simulink model "nonlinearAirframe"  (R2018a)
settings: Solver=ode3  StartTime=0  StopTime=10.0  FixedStep=Ts  RelTol=1e-3  EnableMultiTasking=on
undefined symbols (not defined in the file): e_m_X, e_m_Y, e_p_X, e_p_Y, Earth, initPosLLA, k_ac_X, k_ac_Y, k_as_X, k_as_Y, k_ra_X, k_ra_Y, k_rs_X, k_rs_Y, r_m_X, r_m_Y, r_sm_X, r_sm_Y, Vehicle, WGS84
libraries: actuatorsLibrary x3, shared6dof x1, aerolibtransform2 x1
settings Model: Creator=The MathWorks, Inc.  LastModifiedBy=Ducted Fan
settings SolverCC: AutoInsertRateTranBlk=on
settings DataIOCC: SaveFormat=Array  SaveOutput=off  SignalLogging=off  DSMLogging=off  SaveTime=off
settings OptimizationCC: BlockReduction=off  DefaultParameterBehavior=Inlined  BufferReuse=off  LifeSpan=inf
settings DebuggingCC: AlgebraicLoopMsg=none  UnderspecifiedInitializationDetection=Classic  MergeDetectMultiDrivingBlocksExec=none  UnconnectedInputMsg=none  UnconnectedOutputMsg=none  UnconnectedLineMsg=none  AllowSymbolicDim=off  SFUnexpectedBacktrackingDiag=warning  SFNoUnconditionalDefaultTransitionDiag=warning  SFExecutionAtInitializationDiag=none
settings HardwareCC: ProdBitPerPointer=32  ProdBitPerSizeT=32  ProdBitPerPtrDiffT=32  ProdLargestAtomicFloat=None  ProdIntDivRoundTo=Undefined  ProdEndianess=Unspecified  ProdWordSize=32  ProdHWDeviceType=32-bit Generic
settings ModelReferenceCC: PropagateSignalLabelsOutOfModel=off
settings CodeAppCC: StateflowObjectComments=on
settings GRTTargetCC: TargetLangStandard=C89/C90 (ANSI)  GeneratePreprocessorConditionals=Disable all
settings ConfigComp: CovMetricSettings=dw  CovHtmlReporting=on  CovSaveCumulativeToWorkspaceVar=on  CovSaveSingleToWorkspaceVar=on  CovExternalEMLEnable=off  CovSFcnEnable=off

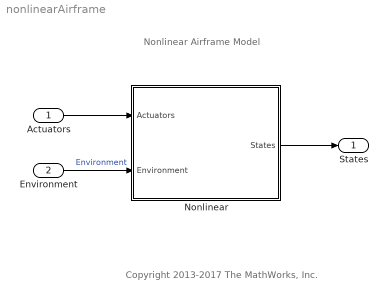
== system nonlinearAirframe ==
  note: Copyright 2013-2017 The MathWorks, Inc.
  note: Nonlinear Airframe Model
  Actuators : Inport  OutDataTypeStr=Bus: ActuatorsBus
  Environment : Inport  Port=2  OutDataTypeStr=Bus: EnvironmentBus  BusOutputAsStruct=on
  Nonlinear : Subsystem  TreatAsAtomicUnit=on
      mask init:
      | vehicleNonlinearVars;
  States : Outport  OutDataTypeStr=Bus: StatesBus  BusOutputAsStruct=on
  wires:
  Actuators/1 -> Nonlinear/1(Actuators)
  Environment/1 -> Nonlinear/2(Environment)  "Environment"
  Nonlinear/1(States) -> States/1

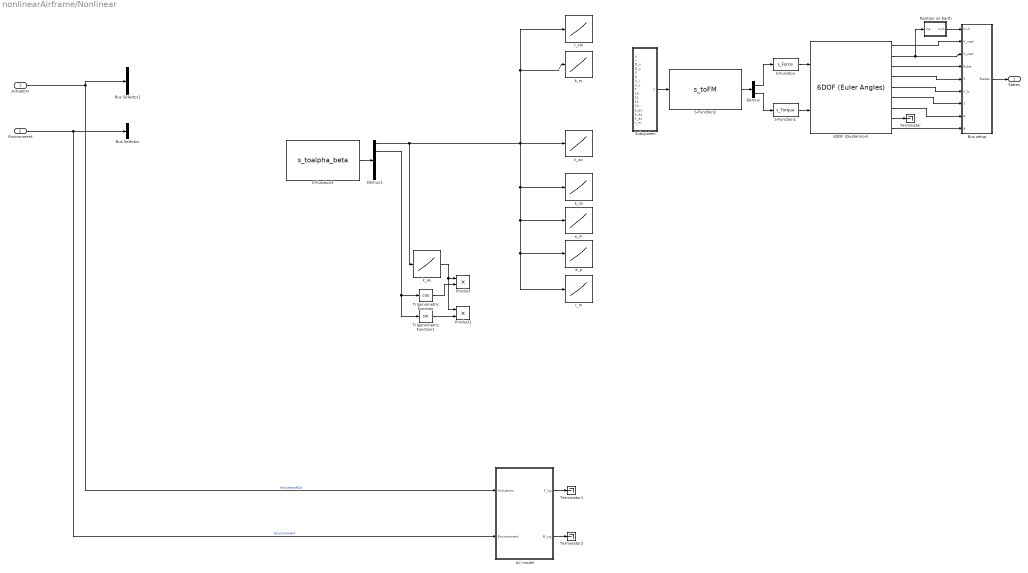
== system nonlinearAirframe/Nonlinear ==
  Actuators : Inport  OutDataTypeStr=Bus: ActuatorsBus
  Environment : Inport  Port=2  OutDataTypeStr=Bus: EnvironmentBus
  6DOF (Quaternion) : shared6dof/6DOF (Euler Angles)  units=Metric (MKS)  mtype=Fixed  rep=Quaternion  xme_0=initPosNED  Vm_0=initVb  eul_0=initEuler  pm_0=initAngRates  mass_0=mass  mass_e=0.5  mass_f=2.0  inertia=inertia  inertia_e=eye(3)  inertia_f=2*eye(3)  k_quat=Vehicle.Nonlinear.Nonlinear.SixDOF.quatGain  vre_flag=on  abi_flag=on  aMode=aMode
      settings: SourceProductBaseCode=AE
  AC model : Subsystem
  Bus Selector : BusSelector  OutputSignals=StatesBus.V_body,StatesBus.DCM_be,WindBus.wind_xy,WindBus.wind_d
  Bus Selector1 : BusSelector  OutputSignals=c1,c2,c3,c4,speed
  Bus setup : Subsystem
  Demux : Demux  Outputs=2
  Demux1 : Demux  Outputs=5
  Position on Earth : Subsystem  Priority=1  TreatAsAtomicUnit=on
  Product : Product
  Product1 : Product
  S-Function : S-Function  FunctionName=s_Force  SFunctionDeploymentMode=off  EnableBusSupport=off
  S-Function1 : S-Function  FunctionName=s_Torque  SFunctionDeploymentMode=off  EnableBusSupport=off
  S-Function2 : S-Function  FunctionName=s_toFM  SFunctionDeploymentMode=off  EnableBusSupport=off
  S-Function3 : S-Function  FunctionName=s_toalpha_beta  SFunctionDeploymentMode=off  EnableBusSupport=off
  Subsystem : Subsystem
  Terminator : Terminator
  Terminator1 : Terminator
  Terminator2 : Terminator
  Trigonometric Function : Trigonometry  Operator=cos
  Trigonometric Function1 : Trigonometry
  e_m : Lookup_n-D  NumberOfTableDimensions=1  BreakpointsForDimension1=e_m_X  Table=e_m_Y  InternalRulePriority=Speed  RndMeth=Simplest  InputSameDT=on
  e_p : Lookup_n-D  NumberOfTableDimensions=1  BreakpointsForDimension1=e_p_X  Table=e_p_Y  InternalRulePriority=Speed  RndMeth=Simplest  InputSameDT=on
  k_ac : Lookup_n-D  NumberOfTableDimensions=1  BreakpointsForDimension1=k_ac_X  Table=k_ac_Y  InternalRulePriority=Speed  RndMeth=Simplest  InputSameDT=on
  k_as : Lookup_n-D  NumberOfTableDimensions=1  BreakpointsForDimension1=k_as_X  Table=k_as_Y  InternalRulePriority=Speed  RndMeth=Simplest  InputSameDT=on
  k_ra : Lookup_n-D  NumberOfTableDimensions=1  BreakpointsForDimension1=k_ra_X  Table=k_ra_Y  InternalRulePriority=Speed  RndMeth=Simplest  InputSameDT=on
  "k_rs " : Lookup_n-D  NumberOfTableDimensions=1  BreakpointsForDimension1=k_rs_X  Table=k_rs_Y  InternalRulePriority=Speed  RndMeth=Simplest  InputSameDT=on
  r_m : Lookup_n-D  NumberOfTableDimensions=1  BreakpointsForDimension1=r_m_X  Table=r_m_Y  InternalRulePriority=Speed  RndMeth=Simplest  InputSameDT=on
  r_sm : Lookup_n-D  NumberOfTableDimensions=1  BreakpointsForDimension1=r_sm_X  Table=r_sm_Y  InternalRulePriority=Speed  RndMeth=Simplest  InputSameDT=on
  States : Outport
  wires:
  6DOF (Quaternion)/1 -> Bus setup/2(V_ned)
  6DOF (Quaternion)/2 -> Position on Earth/1(Xe), Bus setup/3(X_ned)
  6DOF (Quaternion)/3 -> Bus setup/4(Euler)
  6DOF (Quaternion)/4 -> Bus setup/5(DCM_be)
  6DOF (Quaternion)/5 -> Bus setup/6(V_b)
  6DOF (Quaternion)/6 -> Bus setup/7(Omega_b)
  6DOF (Quaternion)/7 -> Bus setup/8(dOmega_b)
  Position on Earth/1(LLA) -> Bus setup/1(LLA)
  Bus setup/1(States) -> States/1
  6DOF (Quaternion)/9 -> Bus setup/9(Accel_b)
  6DOF (Quaternion)/8 -> Terminator/1
  AC model/1(F_cg) -> Terminator1/1
  AC model/2(M_cg) -> Terminator2/1
  S-Function1/1 -> 6DOF (Quaternion)/2
  S-Function/1 -> 6DOF (Quaternion)/1
  Actuators/1 -> Bus Selector1/1, AC model/1(Actuators)  "ActuatorsBus"
  Environment/1 -> Bus Selector/1, AC model/2(Environment)  "Environment"
  Subsystem/1(Out1) -> S-Function2/1
  S-Function2/1 -> Demux/1
  Demux/1 -> S-Function/1
  Demux/2 -> S-Function1/1
  S-Function3/1 -> Demux1/1
  Demux1/1 -> "k_rs "/1, r_sm/1, k_ra/1, e_m/1, e_p/1, r_m/1, k_ac/1, k_as/1
  Demux1/2 -> Trigonometric Function/1, Trigonometric Function1/1
  k_as/1 -> Product1/1, Product/1
  Trigonometric Function/1 -> Product/2
  Trigonometric Function1/1 -> Product1/2

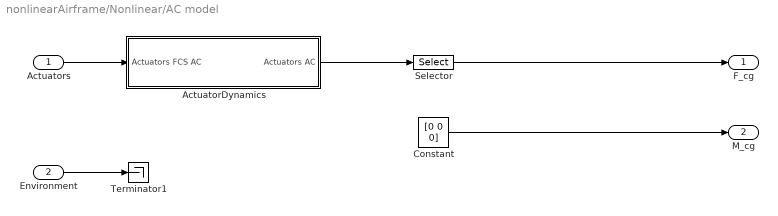
== system nonlinearAirframe/Nonlinear/AC model ==
  Actuators : Inport
  Environment : Inport  Port=2
  ActuatorDynamics : Subsystem  Variant=on
  Constant : Constant  Value=[0 0 0]
  Selector : Selector  InputPortWidth=4  IndexOptions=Index vector (dialog)  Indices=[1 2 3]  OutputSizes=1
  Terminator1 : Terminator
  F_cg : Outport
  M_cg : Outport  Port=2
  wires:
  Environment/1 -> Terminator1/1
  Selector/1 -> F_cg/1
  Actuators/1 -> ActuatorDynamics/1(Actuators FCS AC)
  ActuatorDynamics/1(Actuators AC) -> Selector/1
  Constant/1 -> M_cg/1

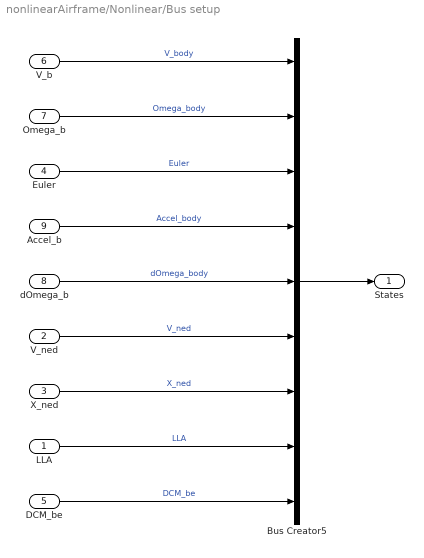
== system nonlinearAirframe/Nonlinear/Bus setup ==
  LLA : Inport  PortDimensions=3
  V_ned : Inport  Port=2  PortDimensions=3
  X_ned : Inport  Port=3  PortDimensions=3
  Euler : Inport  Port=4  PortDimensions=3
  DCM_be : Inport  Port=5  PortDimensions=[3 3]
  V_b : Inport  Port=6  PortDimensions=3
  Omega_b : Inport  Port=7  PortDimensions=3
  dOmega_b : Inport  Port=8  PortDimensions=3
  Accel_b : Inport  Port=9  PortDimensions=3
  Bus Creator5 : BusCreator  Inputs=9  OutDataTypeStr=Bus: StatesBus  NonVirtualBus=on
  States : Outport
  wires:
  Bus Creator5/1 -> States/1
  V_b/1 -> Bus Creator5/1  "V_body"
  Omega_b/1 -> Bus Creator5/2  "Omega_body"
  Euler/1 -> Bus Creator5/3  "Euler"
  X_ned/1 -> Bus Creator5/7  "X_ned"
  Accel_b/1 -> Bus Creator5/4  "Accel_body"
  LLA/1 -> Bus Creator5/8  "LLA"
  dOmega_b/1 -> Bus Creator5/5  "dOmega_body"
  DCM_be/1 -> Bus Creator5/9  "DCM_be"
  V_ned/1 -> Bus Creator5/6  "V_ned"

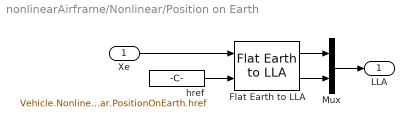
== system nonlinearAirframe/Nonlinear/Position on Earth ==
  Xe : Inport
  Flat Earth to LLA : aerolibtransform2/Flat Earth to LLA  units=Metric (MKS)  ptype=Earth (WGS84)  F=1/298.257223563  R=6378137  LL0=initPosLLA(1:2)  psi=Vehicle.Nonlinear.Nonlinear.PositionOnEarth.FlatEarthToLLA.xAxis
  Mux : Mux  Inputs=2
  href : Constant  Value=Vehicle.Nonlinear.Nonlinear.PositionOnEarth.href
  LLA : Outport
  wires:
  Mux/1 -> LLA/1
  Xe/1 -> Flat Earth to LLA/1
  Flat Earth to LLA/1 -> Mux/1
  Flat Earth to LLA/2 -> Mux/2
  href/1 -> Flat Earth to LLA/2

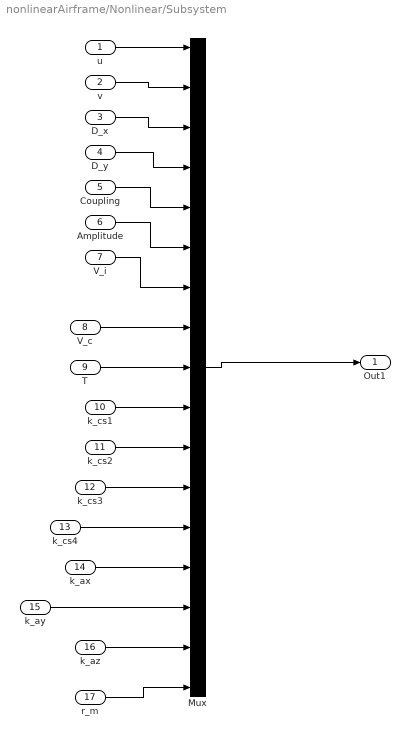
== system nonlinearAirframe/Nonlinear/Subsystem ==
  u : Inport
  v : Inport  Port=2
  D_x : Inport  Port=3
  D_y : Inport  Port=4
  Coupling : Inport  Port=5
  Amplitude : Inport  Port=6
  V_i : Inport  Port=7
  V_c : Inport  Port=8
  T : Inport  Port=9
  k_cs1 : Inport  Port=10
  k_cs2 : Inport  Port=11
  k_cs3 : Inport  Port=12
  k_cs4 : Inport  Port=13
  k_ax : Inport  Port=14
  k_ay : Inport  Port=15
  k_az : Inport  Port=16
  r_m : Inport  Port=17
  Mux : Mux  Inputs=17
  Out1 : Outport
  wires:
  u/1 -> Mux/1
  v/1 -> Mux/2
  D_x/1 -> Mux/3
  D_y/1 -> Mux/4
  Coupling/1 -> Mux/5
  Amplitude/1 -> Mux/6
  V_i/1 -> Mux/7
  V_c/1 -> Mux/8
  T/1 -> Mux/9
  k_cs1/1 -> Mux/10
  k_cs2/1 -> Mux/11
  k_cs3/1 -> Mux/12
  k_cs4/1 -> Mux/13
  k_ax/1 -> Mux/14
  k_ay/1 -> Mux/15
  k_az/1 -> Mux/16
  Mux/1 -> Out1/1
  r_m/1 -> Mux/17

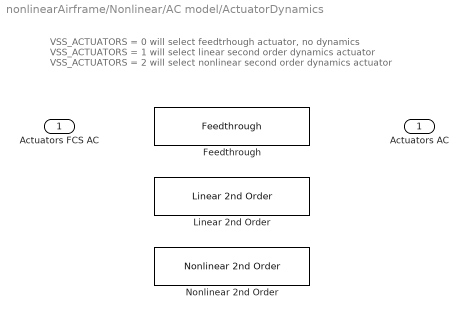
== system nonlinearAirframe/Nonlinear/AC model/ActuatorDynamics ==
  note: VSS_ACTUATORS = 0 will select feedtrhough actuator, no dynamics
      | VSS_ACTUATORS = 1 will select linear second order dynamics actuator
      | VSS_ACTUATORS = 2 will select nonlinear second order dynamics actuator
  Actuators FCS AC : Inport
  Feedthrough : actuatorsLibrary/Feedthrough  VariantControl=VSS_ACTUATORS_FEEDTHROUGH
  Linear 2nd Order : actuatorsLibrary/Linear 2nd Order  VariantControl=VSS_ACTUATORS_LINEAR
  Nonlinear 2nd Order : actuatorsLibrary/Nonlinear 2nd Order  VariantControl=VSS_ACTUATORS_NONLINEAR
  Actuators AC : Outport
